simulink model "DC_DC_buck_Microgrid_sim_4"  (R2015a)
settings: Solver=ode23tb  StartTime=0.0  StopTime=0.05  MaxStep=1/fpwm/200  RelTol=1e-3
values from neighbouring files (symbols this model uses):
  Cf = 2*IoAVmin/(8*fpwm*DeltaVo*Vo)    (= 5.42534722222e-05)    [DC_DC_buck_Microgrid_1_2_3.m]    (also in DC_DC_buck_Microgrid_4.m = 2.71267361111e-05)
  Cf2 = 2*IoAVmin2/(8*fpwm2*DeltaVo2*Vo2)    (= 5.42534722222e-05)    [DC_DC_buck_Microgrid_4.m]
  deltaN = Vo/U    (= 0.48)    [DC_DC_buck_Microgrid_1_2_3.m]    (also in DC_DC_buck_Microgrid_4.m)
  fpwm = 10000    [DC_DC_buck_Microgrid_1_2_3.m]    (also in DC_DC_buck_Microgrid_4.m = 20000)
  fpwm2 = 10000    [DC_DC_buck_Microgrid_4.m]
  IoAVmin = Pomin/Vo    (= 2.08333333333)    [DC_DC_buck_Microgrid_1_2_3.m]    (also in DC_DC_buck_Microgrid_4.m)
  IoAVmin2 = Pomin2/Vo2    (= 2.08333333333)    [DC_DC_buck_Microgrid_4.m]
  Ios = (Pom-Pp-Pomin-Vo^2/Reqp)/Vo    [DC_DC_buck_Microgrid_1_2_3.m]    (also in DC_DC_buck_Microgrid_4.m = 15.625)
  kdv = -(Vomin-Vomax)/(Po-Pomin)    (= 0.00571428571429)    [DC_DC_buck_Microgrid_4.m]
  kdv2 = -(Vomin2-Vomax2)/(Po2-Pomin2)    (= 0.00333333333333)    [DC_DC_buck_Microgrid_4.m]
  Ki = 1/Tp    (= 153.646401213)    [DC_DC_buck_Microgrid_1_2_3.m]    (also in DC_DC_buck_Microgrid_4.m = 307.292802426)
  Ki2 = 1/Tp2    (= 76.8232006066)    [DC_DC_buck_Microgrid_4.m]
  Kiv = 1/Tpv    (= 2252.73933103)    [DC_DC_buck_Microgrid_1_2_3.m]    (also in DC_DC_buck_Microgrid_4.m = 4505.47866205)
  Kiv2 = 1/Tpv2    (= 3754.56555171)    [DC_DC_buck_Microgrid_4.m]
  Kp = Tz/Tp    (= 0.0678081650224)    [DC_DC_buck_Microgrid_1_2_3.m]    (also in DC_DC_buck_Microgrid_4.m)
  Kp2 = Tz2/Tp2    (= 0.0632538852821)    [DC_DC_buck_Microgrid_4.m]
  Kpv = Tzv/Tpv    (= 0.187728277586)    [DC_DC_buck_Microgrid_1_2_3.m]    (also in DC_DC_buck_Microgrid_4.m)
  Kpv2 = Tzv2/Tpv2    (= 0.187728277586)    [DC_DC_buck_Microgrid_4.m]
  Lf = 1.01*Vo*(1-deltamin)/(2*IoAVmin*fpwm)    (= 0.000677876869565)    [DC_DC_buck_Microgrid_1_2_3.m]    (also in DC_DC_buck_Microgrid_4.m = 0.000338938434783)
  Lf2 = 1.01*Vo2*(1-deltamin2)/(2*IoAVmin2*fpwm2)    (= 0.000758817391304)    [DC_DC_buck_Microgrid_4.m]
  Po = 1500    [DC_DC_buck_Microgrid_1_2_3.m]    (also in DC_DC_buck_Microgrid_4.m)
  Po2 = 2500    [DC_DC_buck_Microgrid_4.m]
  Pomin = 100    [DC_DC_buck_Microgrid_1_2_3.m]    (also in DC_DC_buck_Microgrid_4.m)
  Pomin2 = 100    [DC_DC_buck_Microgrid_4.m]
  Rdv = -(Vomin-Vomax)/(Imax-Imin)    (= 0.274285714286)    [DC_DC_buck_Microgrid_4.m]
  Rdv2 = -(Vomin2-Vomax2)/(Imax2-Imin2)    (= 0.16)    [DC_DC_buck_Microgrid_4.m]
  Req = Vo^2/Po    (= 1.536)    [DC_DC_buck_Microgrid_1_2_3.m]    (also in DC_DC_buck_Microgrid_4.m = 1.64571428571)
  Req2 = Vomin2^2/(Po2-Pomin2)    (= 0.96)    [DC_DC_buck_Microgrid_4.m]
  ri = 0.01    [DC_DC_buck_Microgrid_1_2_3.m]    (also in DC_DC_buck_Microgrid_4.m)
  ri2 = 0.005    [DC_DC_buck_Microgrid_4.m]
  rLine = 0.04    [DC_DC_buck_Microgrid_4.m]
  rLine2 = 0.04    [DC_DC_buck_Microgrid_4.m]
  Rmax = Vo^2/Pomin    (= 23.04)    [DC_DC_buck_Microgrid_1_2_3.m]    (also in DC_DC_buck_Microgrid_4.m)
  Rmax2 = Vo2^2/Pomin2    (= 23.04)    [DC_DC_buck_Microgrid_4.m]
  U = 100    [DC_DC_buck_Microgrid_1_2_3.m]    (also in DC_DC_buck_Microgrid_4.m)
  U2 = 120    [DC_DC_buck_Microgrid_4.m]
  ucmax = 1    [DC_DC_buck_Microgrid_1_2_3.m]    (also in DC_DC_buck_Microgrid_4.m)
  ucmax2 = 1    [DC_DC_buck_Microgrid_4.m]
  Vo = 48    [DC_DC_buck_Microgrid_1_2_3.m]    (also in DC_DC_buck_Microgrid_4.m)
  Vomax = 56    [DC_DC_buck_Microgrid_4.m]
  Vomin = Vo    (= 48)    [DC_DC_buck_Microgrid_4.m]
  Vomin2 = Vo    (= 48)    [DC_DC_buck_Microgrid_4.m]
libraries: powerlib x39, simulink x5, powerlib_meascontrol x4
settings Model: Creator=fern  LastModifiedBy=fern

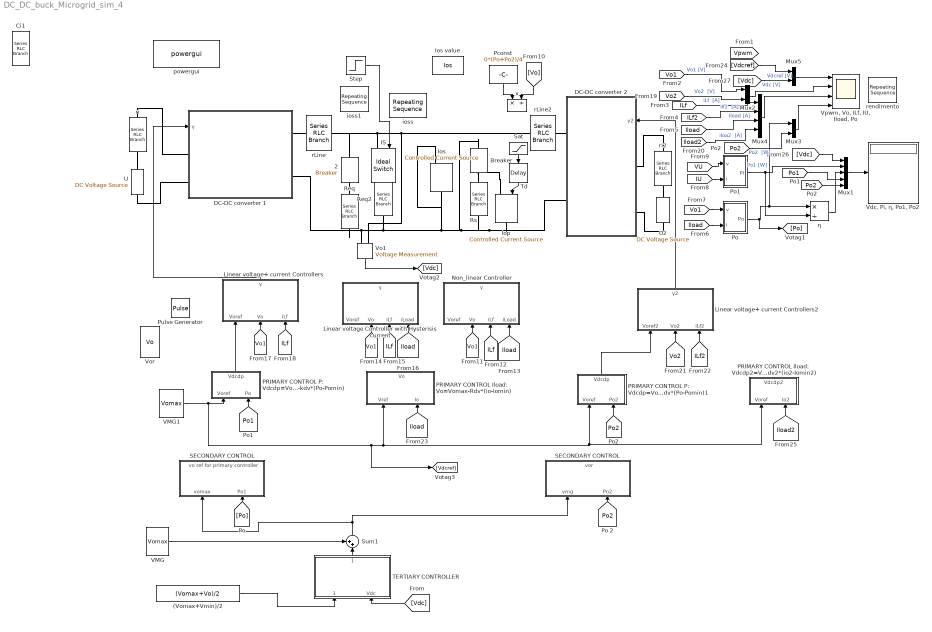
== system DC_DC_buck_Microgrid_sim_4 ==
  (Vomax+Vmin)/2 : Constant  Value=(Vomax+Vo)/2
  2 : powerlib/Elements/Breaker  InitialState=0  SwitchingTimes=[0.01]  External=off  BreakerResistance=0.01  SnubberResistance=Rs  SnubberCapacitance=Cs  Measurements=None  MoreParameters=on  NoBreakLoop=off
  Breaker : powerlib/Elements/Breaker  InitialState=0  SwitchingTimes=[0.04]  External=off  BreakerResistance=0.01  SnubberResistance=Rs  SnubberCapacitance=Cs  Measurements=None  MoreParameters=on  NoBreakLoop=off
  Ci1 : powerlib/Elements/Series RLC Branch  LConnTagsString=__new0  RConnTagsString=__new0  BranchType=C  Resistance=ri  Inductance=1e-6  SetiL0=off  InitialCurrent=4  Capacitance=100e-6  Setx0=on  InitialVoltage=U  Measurements=None
  DC-DC converter 1 : Subsystem
  DC-DC converter 2 : Subsystem
  IS : powerlib/Power Electronics/Ideal Switch  Ron=0.01  Lon=0  IC=0  Rs=Rs  Cs=Cs  Measurements=off
  Iop : powerlib/Electrical Sources/Controlled Current Source  Initialize=on  Source_Type=DC  Amplitude=0  Phase=0  Frequency=0  Measurements=None
  Ios : powerlib/Electrical Sources/Controlled Current Source  Initialize=on  Source_Type=DC  Amplitude=0  Phase=0  Frequency=0  Measurements=None
  Ios value : Constant  Value=Ios
  Linear voltage Controller with Hysterisis current : Subsystem
  Linear voltage+ current Controllers : Subsystem
  Linear voltage+ current Controllers2 : Subsystem
  Mux1 : Mux  Inputs=5
  Mux2 : Mux  Inputs=2
  Mux3 : Mux  Inputs=2
  Mux4 : Mux
  Mux5 : Mux  Inputs=2
  Non_linear Controller : Subsystem
  PRIMARY CONTROL Iload: Vdcdp2=Vomax2-Rdv2*(io2-Iomin2) : Subsystem
  PRIMARY CONTROL Iload: Vo=Vomax-Rdv*(io-Iomin) : Subsystem
  PRIMARY CONTROL P: Vdcdp=Vomax-kdv*(Po-Pomin) : Subsystem
  PRIMARY CONTROL P: Vdcdp=Vomax-kdv*(Po-Pomin)1 : Subsystem
  Pconst : Constant  Value=0*(Po+Po2)/4
  Po : Subsystem
  Po1 : Subsystem
  Pulse Generator : DiscretePulseGenerator  PulseType=Time based  Period=1/fpwm  PulseWidth=deltaN*100
  Req : powerlib/Elements/Series RLC Branch  LConnTagsString=__new0  RConnTagsString=__new0  BranchType=R  Resistance=Req  Inductance=500e-3  SetiL0=on  InitialCurrent=43  Capacitance=[]  Setx0=off  InitialVoltage=0  Measurements=None
  Req2 : powerlib/Elements/Series RLC Branch  LConnTagsString=__new0  RConnTagsString=__new0  BranchType=R  Resistance=Req2  Inductance=500e-3  SetiL0=on  InitialCurrent=43  Capacitance=[]  Setx0=off  InitialVoltage=0  Measurements=None
  Rs : powerlib/Elements/Series RLC Branch  LConnTagsString=__new0  RConnTagsString=__new0  BranchType=R  Resistance=1000*Rmax  Inductance=500e-3  SetiL0=on  InitialCurrent=43  Capacitance=[]  Setx0=off  InitialVoltage=0  Measurements=None
  "SECONDARY CONTROL " : Subsystem
  "SECONDARY CONTROL  " : Subsystem
  Sat : Saturate  UpperLimit=30  LowerLimit=0
  Step : Step  Time=0.02  SampleTime=0
  Sum1 : Sum  Inputs=++|
  TERTIARY CONTROLLER : Subsystem
  Td : TransportDelay  DelayTime=1/(2*fpwm)  BufferSize=2048
  U : powerlib/Electrical Sources/DC Voltage Source  Description=source block  Amplitude=U  Measurements=None
      settings: AttributesFormatString=\n
  U2 : powerlib/Electrical Sources/DC Voltage Source  Description=source block  Amplitude=U2  Measurements=None
      settings: AttributesFormatString=\n
  VMG : Constant  Value=Vomax
  VMG1 : Constant  Value=Vomax
  "Vdc, Pi, η, Po1, Po2" : Display
      settings: Decimation=1000
  Vo1 : powerlib/Measurements/Voltage Measurement  Tag=PoWeRsYsTeMmEaSuReMeNt  PhasorSimulation=off  OutputType=Complex  PSBequivalent=0
  Vor : Constant  Value=Vo
  "Vpwm, Vo, ILf, IU, Iload, Po" : Scope  NumInputPorts=4
      settings: ShowLegends=on  TimeRange=0.0001950120476463327  YMin=55.4~55.3~0~125  YMax=56.3~56.3~5~145  SaveName=psbconverter_str  SampleTime=1/50/512
  ioss : simulink/Sources/Repeating Sequence  rep_seq_t="[0 0.01  0.09 0.1]"  rep_seq_y=[0 0 (Po+Po2-Pomin-Pomin2)/Vomin (Po+Po2-Pomin-Pomin2)/Vomin]
  ioss1 : simulink/Sources/Repeating Sequence  rep_seq_t="[0 0.0149 0.015  0.035 0.03501 0.1]"  rep_seq_y=[0 0 1 1 0 0]
  powergui : powerlib/powergui  Priority=2  SimulationMode=Continuous  SolverType=Tustin/Backward Euler (TBE)  SampleTime=0  frequency=60  SPID=off  DisableSnubberDevices=off  DisableRonSwitches=off  DisableVfSwitches=off  SwTol=0  DisplayEquations=off  Interpol=off  methode=off  Ts=0  FunctionMessages=off  echomessages=off  HookPort=off  EnableUseOfTLC=off  x0status=blocks  frequencyindice=0  Pbase=100e6  ErrMax=1e-4  Iterations=50  UnitsV=kV  UnitsW=MW  buscounter=0  RestoreLinks=warning  ResistiveCurrentMeasurement=off  Frange=[0:2:500]  Ylog=off  Xlog=on  ShowGrid=off  save=off  variable=ZData  structure=psbconverter_str  ZoomFFT=on  StartTime=0.1-2/60  cycles=2  DisplayStyle=off  fundamental=60  FreqAxis=on  MaxFrequency=2000  frequencyindicesteady=1  RmsSteady=1  display=off
  rLine : powerlib/Elements/Series RLC Branch  LConnTagsString=__new0  RConnTagsString=__new0  BranchType=R  Resistance=rLine  Inductance=1e-6  SetiL0=off  InitialCurrent=4  Capacitance=[]  Setx0=off  InitialVoltage=0  Measurements=None
  rLine2 : powerlib/Elements/Series RLC Branch  LConnTagsString=__new0  RConnTagsString=__new0  BranchType=R  Resistance=rLine2  Inductance=1e-6  SetiL0=off  InitialCurrent=4  Capacitance=[]  Setx0=off  InitialVoltage=0  Measurements=None
  rendimento : simulink/Sources/Repeating Sequence  rep_seq_t=[0 0.1]  rep_seq_y=[0 30]
  ri : powerlib/Elements/Series RLC Branch  LConnTagsString=__new0  RConnTagsString=__new0  BranchType=R  Resistance=ri  Inductance=1e-6  SetiL0=off  InitialCurrent=4  Capacitance=[]  Setx0=off  InitialVoltage=0  Measurements=None
  ri2 : powerlib/Elements/Series RLC Branch  LConnTagsString=__new0  RConnTagsString=__new0  BranchType=R  Resistance=ri2  Inductance=1e-6  SetiL0=off  InitialCurrent=4  Capacitance=[]  Setx0=off  InitialVoltage=0  Measurements=None
  x : Product  Inputs=*/
  η : Product  Inputs=*/
  wires:
  Pconst/1 -> x/1
  Mux2/1 -> "Vpwm, Vo, ILf, IU, Iload, Po"/2
  [ILf] -> Mux4/1  "iLf  [A]"
  [Iload] -> Mux4/3  "Iload [A]"
  Mux4/1 -> "Vpwm, Vo, ILf, IU, Iload, Po"/3
  [Vo1] -> Po/1(v)
  [Iload] -> Po/2(i)
  Po/1(Po) -> [Po], Mux3/1, η/1  "Po1 [W]"
  Mux1/1 -> "Vdc, Pi, η, Po1, Po2"/1
  [VU] -> Po1/1(v)
  [IU] -> Po1/2(i)
  Po1/1(Pi) -> η/2, Mux1/2
  [Vo] -> x/2
  Sat/1 -> Td/1
  [Iload] -> Linear voltage Controller with Hysterisis current/4(iLoad)
  [ILf] -> Linear voltage Controller with Hysterisis current/3(iLf)
  [Vo1] -> Linear voltage Controller with Hysterisis current/2(Vo)
  [Vo1] -> Non_linear Controller/2(Vo)
  [ILf] -> Non_linear Controller/3(iLf)
  [Iload] -> Non_linear Controller/4(iLoad)
  [ILf] -> Linear voltage+ current Controllers/3(iLf)
  [Vo1] -> Linear voltage+ current Controllers/2(Vo)
  [Vo1] -> Mux2/1  "Vo1 [V]"
  Mux3/1 -> "Vpwm, Vo, ILf, IU, Iload, Po"/4
  [Vo2] -> Linear voltage+ current Controllers2/2(Vo2)
  [ILf2] -> Linear voltage+ current Controllers2/3(iLf2)
  [Po2] -> PRIMARY CONTROL P: Vdcdp=Vomax-kdv*(Po-Pomin)1/2(Po2)
  [Po1] -> PRIMARY CONTROL P: Vdcdp=Vomax-kdv*(Po-Pomin)/2(Po)
  [Iload] -> PRIMARY CONTROL Iload: Vo=Vomax-Rdv*(io-Iomin)/2(Io)
  Vo1/1 -> [Vdc]
  η/1 -> Mux1/3
  [Po2] -> Mux1/5
  [Po1] -> Mux1/4
  [Iload2] -> PRIMARY CONTROL Iload: Vdcdp2=Vomax2-Rdv2*(io2-Iomin2)/2(Io2)
  [Po] -> "SECONDARY CONTROL "/2(Po1)
  [Po2] -> "SECONDARY CONTROL  "/2(Po2)
  (Vomax+Vmin)/2/1 -> TERTIARY CONTROLLER/1((Vomax+Vmin)/2)
  [Vdc] -> TERTIARY CONTROLLER/2(Vdc)
  Td/1 -> Iop/1
  [Vdc] -> Mux1/1
  Step/1 -> IS/1
  VMG/1 -> Sum1/1
  Mux5/1 -> "Vpwm, Vo, ILf, IU, Iload, Po"/1
  [Vdcref] -> Mux5/1  "Vdcref [V]"
  [Vdc] -> Mux5/2  "Vdc [V]"
  TERTIARY CONTROLLER/1(Voref for secondary controller) -> Sum1/2
  Linear voltage+ current Controllers/1(γ) -> DC-DC converter 1/1(γ)
  Linear voltage+ current Controllers2/1(γ2) -> DC-DC converter 2/1(γ2)
  Sum1/1 -> "SECONDARY CONTROL "/1(vomax), "SECONDARY CONTROL  "/1(vmg)
  [Vo2] -> Mux2/2  "Vo2  [V]"
  [ILf2] -> Mux4/2  "ilf2  [A]"
  [Iload2] -> Mux4/4  "iloa2  [A]"
  [Po2] -> Mux3/2  "Po2  [W]"
  VMG1/1 -> [Vdcref], PRIMARY CONTROL Iload: Vo=Vomax-Rdv*(io-Iomin)/1(Vref), PRIMARY CONTROL Iload: Vdcdp2=Vomax2-Rdv2*(io2-Iomin2)/1(Voref), PRIMARY CONTROL P: Vdcdp=Vomax-kdv*(Po-Pomin)1/1(Voref), PRIMARY CONTROL P: Vdcdp=Vomax-kdv*(Po-Pomin)/1(Voref)
  PRIMARY CONTROL P: Vdcdp=Vomax-kdv*(Po-Pomin)1/1(Vdcdp) -> Linear voltage+ current Controllers2/1(Voref2)
  PRIMARY CONTROL P: Vdcdp=Vomax-kdv*(Po-Pomin)/1(Vdcdp) -> Linear voltage+ current Controllers/1(Voref)
  connections:
  U/RConn1 -- ri/RConn1
  rLine2/RConn1 -- Vo1/LConn1 -- 2/LConn1 -- rLine/RConn1 -- IS/LConn1
  rLine2/LConn1 -- DC-DC converter 2/RConn1
  2/RConn1 -- Req/LConn1
  IS/RConn1 -- Req2/LConn1
  Rs/LConn1 -- Breaker/RConn1 -- Iop/LConn1
  Req2/RConn1 -- Breaker/LConn1 -- DC-DC converter 2/RConn2 -- Iop/RConn1 -- Rs/RConn1 -- Ios/LConn1 -- Ios/RConn1 -- Vo1/LConn2 -- DC-DC converter 1/RConn2 -- Req/RConn1
  DC-DC converter 1/LConn1 -- ri/LConn1
  DC-DC converter 1/LConn2 -- U/LConn1
  DC-DC converter 1/RConn1 -- rLine/LConn1
  U2/RConn1 -- ri2/RConn1
  ri2/LConn1 -- DC-DC converter 2/LConn1
  U2/LConn1 -- DC-DC converter 2/LConn2

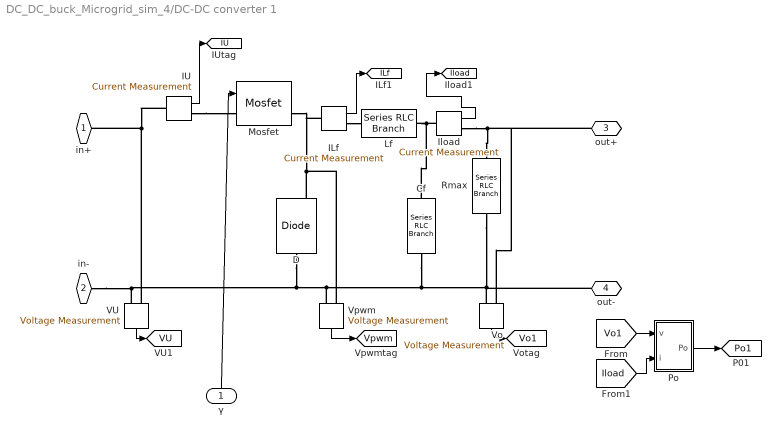
== system DC_DC_buck_Microgrid_sim_4/DC-DC converter 1 ==
  γ : Inport
  Cf : powerlib/Elements/Series RLC Branch  LConnTagsString=__new0  RConnTagsString=__new0  BranchType=C  Resistance=ri  Inductance=Lf  SetiL0=on  InitialCurrent=IoAVmin  Capacitance=Cf  Setx0=on  InitialVoltage=Vo  Measurements=None
  D : powerlib/Power Electronics/Diode  Ron=Ron  Lon=0  Vf=Vd  IC=0  UseSnubber=off  Rs=Rs  Cs=Cs  Measurements=on
  ILf : powerlib/Measurements/Current Measurement  PhasorSimulation=off  OutputType=Complex  PSBequivalent=0
  IU : powerlib/Measurements/Current Measurement  PhasorSimulation=off  OutputType=Complex  PSBequivalent=0
  Iload : powerlib/Measurements/Current Measurement  PhasorSimulation=off  OutputType=Complex  PSBequivalent=0
  Lf : powerlib/Elements/Series RLC Branch  LConnTagsString=__new0  RConnTagsString=__new0  BranchType=L  Resistance=ri  Inductance=Lf  SetiL0=on  InitialCurrent=IoAVmin  Capacitance=[]  Setx0=off  InitialVoltage=0  Measurements=None
  Mosfet : powerlib/Power Electronics/Mosfet  Ron=Rdson  Lon=0  Rd=Rdson  Vfd=0  IC=0  Rs=Rs  Cs=Cs  Measurements=on
  Po : Subsystem
  Rmax : powerlib/Elements/Series RLC Branch  LConnTagsString=__new0  RConnTagsString=__new0  BranchType=R  Resistance=Rmax  Inductance=500e-3  SetiL0=on  InitialCurrent=43  Capacitance=[]  Setx0=off  InitialVoltage=0  Measurements=None
  VU : powerlib/Measurements/Voltage Measurement  Tag=PoWeRsYsTeMmEaSuReMeNt  PhasorSimulation=off  OutputType=Complex  PSBequivalent=0
  Vo : powerlib/Measurements/Voltage Measurement  Tag=PoWeRsYsTeMmEaSuReMeNt  PhasorSimulation=off  OutputType=Complex  PSBequivalent=0
  Vpwm : powerlib/Measurements/Voltage Measurement  Tag=PoWeRsYsTeMmEaSuReMeNt  PhasorSimulation=off  OutputType=Complex  PSBequivalent=0
  in+ : PMIOPort  Port=1  Side=Left
  in- : PMIOPort  Port=2  Side=Left
  out+ : PMIOPort  Port=3  Side=Right
  out- : PMIOPort  Port=4  Side=Right
  tag scope: ILf=global, IU=global, Iload=global, Po1=global, VU=global, Vo1=global, Vpwm=global
  wires:
  Iload/1 -> [Iload]
  Vo/1 -> [Vo1]
  Vpwm/1 -> [Vpwm]
  IU/1 -> [IU]
  VU/1 -> [VU]
  ILf/1 -> [ILf]
  γ/1 -> Mosfet/1
  [Vo1] -> Po/1(v)
  [Iload] -> Po/2(i)
  Po/1(Po) -> [Po1]
  connections:
  VU/LConn2 -- D/LConn1 -- Vpwm/LConn2 -- Cf/RConn1 -- out-/RConn1 -- Vo/LConn2 -- Rmax/RConn1 -- in-/RConn1
  D/RConn1 -- Mosfet/RConn1 -- ILf/LConn1 -- Vpwm/LConn1
  VU/LConn1 -- IU/LConn1 -- in+/RConn1
  Cf/LConn1 -- Iload/LConn1 -- Lf/RConn1
  ILf/RConn1 -- Lf/LConn1
  IU/RConn1 -- Mosfet/LConn1
  Iload/RConn1 -- out+/RConn1 -- Vo/LConn1 -- Rmax/LConn1

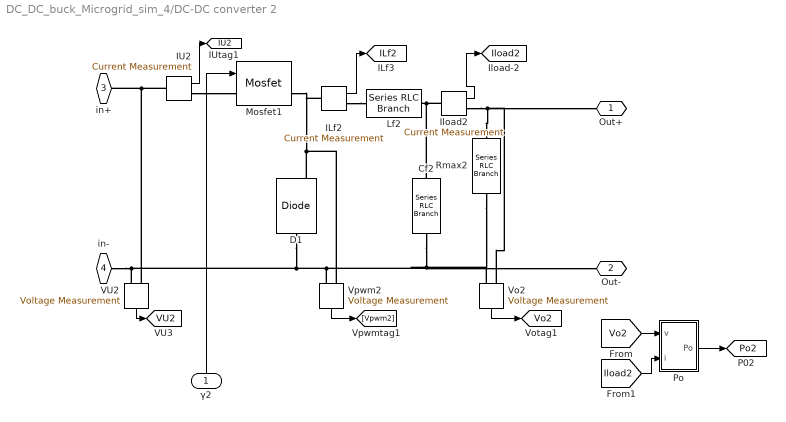
== system DC_DC_buck_Microgrid_sim_4/DC-DC converter 2 ==
  γ2 : Inport
  Cf2 : powerlib/Elements/Series RLC Branch  LConnTagsString=__new0  RConnTagsString=__new0  BranchType=C  Resistance=ri  Inductance=Lf  SetiL0=on  InitialCurrent=IoAVmin  Capacitance=Cf2  Setx0=on  InitialVoltage=Vo  Measurements=None
  D1 : powerlib/Power Electronics/Diode  Ron=Ron2  Lon=0  Vf=Vd2  IC=0  UseSnubber=off  Rs=Rs2  Cs=Cs2  Measurements=on
  ILf2 : powerlib/Measurements/Current Measurement  PhasorSimulation=off  OutputType=Complex  PSBequivalent=0
  IU2 : powerlib/Measurements/Current Measurement  PhasorSimulation=off  OutputType=Complex  PSBequivalent=0
  Iload2 : powerlib/Measurements/Current Measurement  PhasorSimulation=off  OutputType=Complex  PSBequivalent=0
  Lf2 : powerlib/Elements/Series RLC Branch  LConnTagsString=__new0  RConnTagsString=__new0  BranchType=L  Resistance=ri  Inductance=Lf2  SetiL0=off  InitialCurrent=IoAV2min  Capacitance=[]  Setx0=off  InitialVoltage=0  Measurements=None
  Mosfet1 : powerlib/Power Electronics/Mosfet  Ron=Rdson2  Lon=0  Rd=Rdson2  Vfd=0  IC=0  Rs=Rs2  Cs=Cs2  Measurements=on
  Po : Subsystem
  Rmax2 : powerlib/Elements/Series RLC Branch  LConnTagsString=__new0  RConnTagsString=__new0  BranchType=R  Resistance=Rmax2  Inductance=500e-3  SetiL0=on  InitialCurrent=43  Capacitance=[]  Setx0=off  InitialVoltage=0  Measurements=None
  VU2 : powerlib/Measurements/Voltage Measurement  Tag=PoWeRsYsTeMmEaSuReMeNt  PhasorSimulation=off  OutputType=Complex  PSBequivalent=0
  Vo2 : powerlib/Measurements/Voltage Measurement  Tag=PoWeRsYsTeMmEaSuReMeNt  PhasorSimulation=off  OutputType=Complex  PSBequivalent=0
  Vpwm2 : powerlib/Measurements/Voltage Measurement  Tag=PoWeRsYsTeMmEaSuReMeNt  PhasorSimulation=off  OutputType=Complex  PSBequivalent=0
  Out+ : PMIOPort  Port=1  Side=Right
  Out- : PMIOPort  Port=2  Side=Right
  in+ : PMIOPort  Port=3  Side=Left
  in- : PMIOPort  Port=4  Side=Left
  tag scope: ILf2=global, IU2=global, Iload2=global, Po2=global, VU2=global, Vo2=global
  wires:
  VU2/1 -> [VU2]
  IU2/1 -> [IU2]
  Iload2/1 -> [Iload2]
  Vo2/1 -> [Vo2]
  ILf2/1 -> [ILf2]
  γ2/1 -> Mosfet1/1
  Vpwm2/1 -> [Vpwm2]
  [Vo2] -> Po/1(v)
  [Iload2] -> Po/2(i)
  Po/1(Po) -> [Po2]
  connections:
  D1/RConn1 -- Vpwm2/LConn1 -- ILf2/LConn1 -- Mosfet1/RConn1
  D1/LConn1 -- VU2/LConn2 -- in-/RConn1 -- Vpwm2/LConn2 -- Cf2/RConn1 -- Out-/RConn1 -- Vo2/LConn2 -- Rmax2/RConn1
  VU2/LConn1 -- in+/RConn1 -- IU2/LConn1
  Cf2/LConn1 -- Iload2/LConn1 -- Lf2/RConn1
  IU2/RConn1 -- Mosfet1/LConn1
  ILf2/RConn1 -- Lf2/LConn1
  Iload2/RConn1 -- Out+/RConn1 -- Vo2/LConn1 -- Rmax2/LConn1

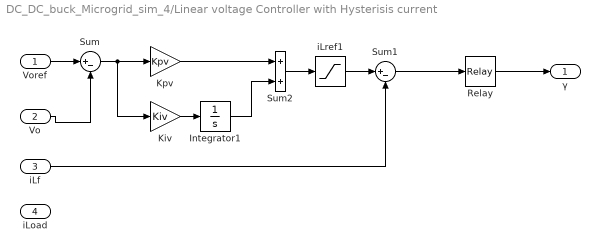
== system DC_DC_buck_Microgrid_sim_4/Linear voltage Controller with Hysterisis current ==
  Voref : Inport
  Vo : Inport  Port=2
  iLf : Inport  Port=3
  iLoad : Inport  Port=4
  Integrator1 : Integrator  LimitOutput=on  UpperSaturationLimit=60  LowerSaturationLimit=-60
  Kiv : Gain  Gain=Kiv
  Kpv : Gain  Gain=Kpv
  Relay : Relay  OnSwitchValue=IoAVmin/2  OffSwitchValue=-IoAVmin/2
  Sum : Sum  Inputs=|+-
  Sum1 : Sum  Inputs=|+-
  Sum2 : Sum
  iLref1 : Saturate  UpperLimit=60  LowerLimit=0
  γ : Outport
  wires:
  Kpv/1 -> Sum2/1
  Sum1/1 -> Relay/1
  Sum/1 -> Kiv/1, Kpv/1
  Vo/1 -> Sum/2
  Voref/1 -> Sum/1
  Relay/1 -> γ/1
  Sum2/1 -> iLref1/1
  iLf/1 -> Sum1/2
  Kiv/1 -> Integrator1/1
  Integrator1/1 -> Sum2/2
  iLref1/1 -> Sum1/1

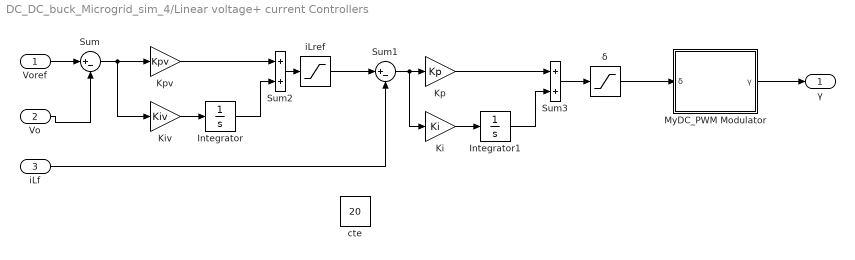
== system DC_DC_buck_Microgrid_sim_4/Linear voltage+ current Controllers ==
  Voref : Inport
  Vo : Inport  Port=2
  iLf : Inport  Port=3
  Integrator : Integrator  LimitOutput=on  UpperSaturationLimit=1.3*Po/Vomin  LowerSaturationLimit=-1.3*Po/Vomin
  Integrator1 : Integrator  LimitOutput=on  UpperSaturationLimit=1  LowerSaturationLimit=-1
  Ki : Gain  Gain=Ki
  Kiv : Gain  Gain=Kiv
  Kp : Gain  Gain=Kp
  Kpv : Gain  Gain=Kpv
  MyDC_PWM Modulator : Subsystem
  Sum : Sum  Inputs=|+-
  Sum1 : Sum  Inputs=|+-
  Sum2 : Sum
  Sum3 : Sum
  cte : Constant  Value=20
  iLref : Saturate  UpperLimit=1.3*Po/Vomin  LowerLimit=0
  δ : Saturate  UpperLimit=0.99  LowerLimit=0.01
  γ : Outport
  wires:
  Integrator/1 -> Sum2/2
  Kiv/1 -> Integrator/1
  iLf/1 -> Sum1/2
  Sum2/1 -> iLref/1
  Voref/1 -> Sum/1
  Vo/1 -> Sum/2
  Sum/1 -> Kpv/1, Kiv/1
  Kpv/1 -> Sum2/1
  Integrator1/1 -> Sum3/2
  Ki/1 -> Integrator1/1
  Sum3/1 -> δ/1
  Sum1/1 -> Kp/1, Ki/1
  Kp/1 -> Sum3/1
  iLref/1 -> Sum1/1
  δ/1 -> MyDC_PWM Modulator/1(δ)
  MyDC_PWM Modulator/1(γ) -> γ/1

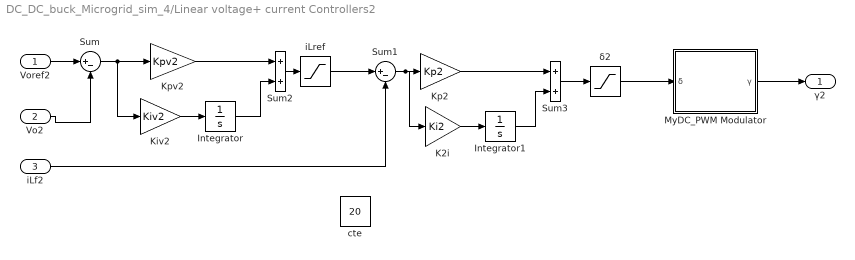
== system DC_DC_buck_Microgrid_sim_4/Linear voltage+ current Controllers2 ==
  Voref2 : Inport
  Vo2 : Inport  Port=2
  iLf2 : Inport  Port=3
  Integrator : Integrator  LimitOutput=on  UpperSaturationLimit=1.3*Po2/Vomin2  LowerSaturationLimit=-1.3*Po2/Vomin2
  Integrator1 : Integrator  LimitOutput=on  UpperSaturationLimit=1  LowerSaturationLimit=-1
  K2i : Gain  Gain=Ki2
  Kiv2 : Gain  Gain=Kiv2
  Kp2 : Gain  Gain=Kp2
  Kpv2 : Gain  Gain=Kpv2
  MyDC_PWM Modulator : Subsystem
  Sum : Sum  Inputs=|+-
  Sum1 : Sum  Inputs=|+-
  Sum2 : Sum
  Sum3 : Sum
  cte : Constant  Value=20
  iLref : Saturate  UpperLimit=1.3*Po2/Vomin2  LowerLimit=0
  δ2 : Saturate  UpperLimit=0.99  LowerLimit=0.01
  γ2 : Outport
  wires:
  MyDC_PWM Modulator/1(γ) -> γ2/1
  δ2/1 -> MyDC_PWM Modulator/1(δ)
  iLref/1 -> Sum1/1
  Kp2/1 -> Sum3/1
  Sum1/1 -> K2i/1, Kp2/1
  Sum3/1 -> δ2/1
  K2i/1 -> Integrator1/1
  Integrator1/1 -> Sum3/2
  Kpv2/1 -> Sum2/1
  Sum/1 -> Kiv2/1, Kpv2/1
  Vo2/1 -> Sum/2
  Voref2/1 -> Sum/1
  Sum2/1 -> iLref/1
  iLf2/1 -> Sum1/2
  Kiv2/1 -> Integrator/1
  Integrator/1 -> Sum2/2

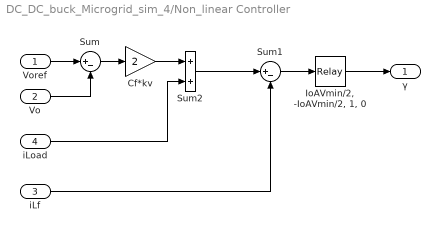
== system DC_DC_buck_Microgrid_sim_4/Non_linear Controller ==
  Voref : Inport
  Vo : Inport  Port=2
  iLf : Inport  Port=3
  iLoad : Inport  Port=4
  Cf*kv : Gain  Gain=2
  "IoAVmin/2, -IoAVmin/2, 1, 0" : Relay  OnSwitchValue=IoAVmin/2  OffSwitchValue=-IoAVmin/2
  Sum : Sum  Inputs=|+-
  Sum1 : Sum  Inputs=|+-
  Sum2 : Sum
  γ : Outport
  wires:
  "IoAVmin/2, -IoAVmin/2, 1, 0"/1 -> γ/1
  Voref/1 -> Sum/1
  Vo/1 -> Sum/2
  Sum/1 -> Cf*kv/1
  iLf/1 -> Sum1/2
  Sum1/1 -> "IoAVmin/2, -IoAVmin/2, 1, 0"/1
  Cf*kv/1 -> Sum2/1
  Sum2/1 -> Sum1/1
  iLoad/1 -> Sum2/2

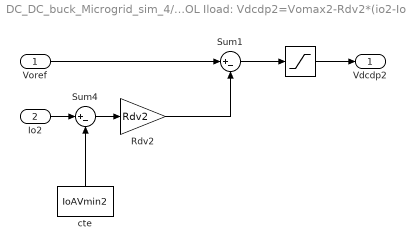
== system DC_DC_buck_Microgrid_sim_4/PRIMARY CONTROL Iload: Vdcdp2=Vomax2-Rdv2*(io2-Iomin2) ==
  Voref : Inport
  Io2 : Inport  Port=2
  " " : Saturate  UpperLimit=Vomax+1  LowerLimit=Vomin-1
  Rdv2 : Gain  Gain=Rdv2
  Sum1 : Sum  Inputs=|+-
  Sum4 : Sum  Inputs=|+-
  cte : Constant  Value=IoAVmin2
  Vdcdp2 : Outport
  wires:
  Sum1/1 -> " "/1
  Voref/1 -> Sum1/1
  Io2/1 -> Sum4/1
  cte/1 -> Sum4/2
  Sum4/1 -> Rdv2/1
  " "/1 -> Vdcdp2/1
  Rdv2/1 -> Sum1/2

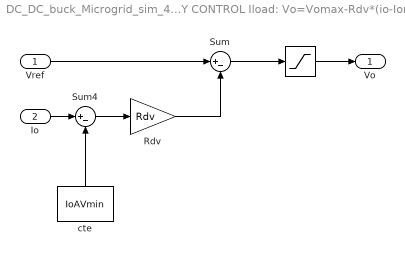
== system DC_DC_buck_Microgrid_sim_4/PRIMARY CONTROL Iload: Vo=Vomax-Rdv*(io-Iomin) ==
  Vref : Inport
  Io : Inport  Port=2
  " " : Saturate  UpperLimit=Vomax+1  LowerLimit=Vomin-1
  Rdv : Gain  Gain=Rdv
  Sum : Sum  Inputs=|+-
  Sum4 : Sum  Inputs=|+-
  cte : Constant  Value=IoAVmin
  Vo : Outport
  wires:
  " "/1 -> Vo/1
  Rdv/1 -> Sum/2
  Sum4/1 -> Rdv/1
  cte/1 -> Sum4/2
  Io/1 -> Sum4/1
  Vref/1 -> Sum/1
  Sum/1 -> " "/1

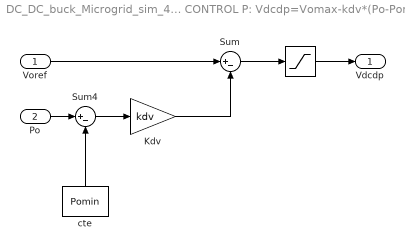
== system DC_DC_buck_Microgrid_sim_4/PRIMARY CONTROL P: Vdcdp=Vomax-kdv*(Po-Pomin) ==
  Voref : Inport
  Po : Inport  Port=2
  " " : Saturate  UpperLimit=Vomax+1  LowerLimit=Vomin-1
  Kdv : Gain  Gain=kdv
  Sum : Sum  Inputs=|+-
  Sum4 : Sum  Inputs=|+-
  cte : Constant  Value=Pomin
  Vdcdp : Outport
  wires:
  Sum/1 -> " "/1
  Voref/1 -> Sum/1
  Po/1 -> Sum4/1
  cte/1 -> Sum4/2
  Sum4/1 -> Kdv/1
  Kdv/1 -> Sum/2
  " "/1 -> Vdcdp/1

== system DC_DC_buck_Microgrid_sim_4/PRIMARY CONTROL P: Vdcdp=Vomax-kdv*(Po-Pomin)1 ==
  Voref : Inport
  Po2 : Inport  Port=2
  " " : Saturate  UpperLimit=Vomax+1  LowerLimit=Vomin-1
  Kdv2 : Gain  Gain=kdv2
  Sum : Sum  Inputs=|+-
  Sum4 : Sum  Inputs=|+-
  cte : Constant  Value=Pomin2
  Vdcdp : Outport
  wires:
  " "/1 -> Vdcdp/1
  Sum4/1 -> Kdv2/1
  cte/1 -> Sum4/2
  Po2/1 -> Sum4/1
  Voref/1 -> Sum/1
  Sum/1 -> " "/1
  Kdv2/1 -> Sum/2

== system DC_DC_buck_Microgrid_sim_4/Po ==
  v : Inport
  i : Inport  Port=2
  Mean : powerlib_meascontrol/Measurements/Mean  Freq=fpwm/10  Vinit=100  Ts=0
  x : Product  Inputs=**
  Po : Outport
  wires:
  x/1 -> Mean/1
  v/1 -> x/1
  i/1 -> x/2
  Mean/1 -> Po/1

== system DC_DC_buck_Microgrid_sim_4/Po1 ==
  v : Inport
  i : Inport  Port=2
  Mean : powerlib_meascontrol/Measurements/Mean  Freq=fpwm/10  Vinit=110  Ts=0
  x : Product  Inputs=**
  Pi : Outport
  wires:
  Mean/1 -> Pi/1
  i/1 -> x/2
  v/1 -> x/1
  x/1 -> Mean/1

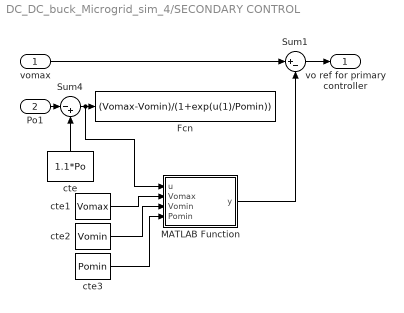
== system DC_DC_buck_Microgrid_sim_4/SECONDARY CONTROL  ==
  vomax : Inport
  Po1 : Inport  Port=2
  Fcn : Fcn  Expr=(Vomax-Vomin)/(1+exp(u(1)/Pomin))
  MATLAB Function : MATLAB Function  TreatAsAtomicUnit=on
  Sum1 : Sum  Inputs=|+-
  Sum4 : Sum  Inputs=|-+
  cte : Constant  Value=1.1*Po
  cte1 : Constant  Value=Vomax
  cte2 : Constant  Value=Vomin
  cte3 : Constant  Value=Pomin
  vo ref for primary controller : Outport
  wires:
  cte/1 -> Sum4/2
  Po1/1 -> Sum4/1
  Sum4/1 -> MATLAB Function/1(u), Fcn/1
  Sum1/1 -> vo ref for primary controller/1
  vomax/1 -> Sum1/1
  cte1/1 -> MATLAB Function/2(Vomax)
  cte2/1 -> MATLAB Function/3(Vomin)
  cte3/1 -> MATLAB Function/4(Pomin)
  MATLAB Function/1(y) -> Sum1/2

== system DC_DC_buck_Microgrid_sim_4/SECONDARY CONTROL   ==
  vmg : Inport
  Po2 : Inport  Port=2
  Fcn : Fcn  Expr=(Vomax-Vomin)/(1+exp(u(1)/Pomin2))
  Sum1 : Sum  Inputs=|+-
  Sum4 : Sum  Inputs=|-+
  cte : Constant  Value=1.1*Po2
  vor : Outport
  wires:
  Sum1/1 -> vor/1
  Po2/1 -> Sum4/1
  cte/1 -> Sum4/2
  Sum4/1 -> Fcn/1
  Fcn/1 -> Sum1/2
  vmg/1 -> Sum1/1

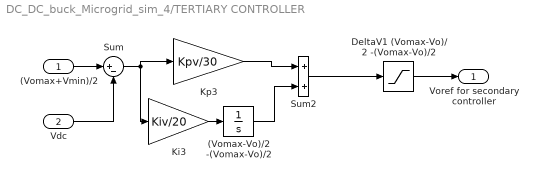
== system DC_DC_buck_Microgrid_sim_4/TERTIARY CONTROLLER ==
  (Vomax+Vmin)/2 : Inport
  Vdc : Inport  Port=2
  (Vomax-Vo)/2 -(Vomax-Vo)/2 : Integrator  LimitOutput=on  UpperSaturationLimit=(Vomax-Vo)/2  LowerSaturationLimit=-(Vomax-Vo)
  DeltaV1 (Vomax-Vo)/2 -(Vomax-Vo)/2 : Saturate  UpperLimit=(Vomax-Vo)/2  LowerLimit=-(Vomax-Vo)/2
  Ki3 : Gain  Gain=Kiv/20
  Kp3 : Gain  Gain=Kpv/30
  Sum : Sum  Inputs=|+-
  Sum2 : Sum
  Voref for secondary controller : Outport
  wires:
  DeltaV1 (Vomax-Vo)/2 -(Vomax-Vo)/2/1 -> Voref for secondary controller/1
  (Vomax-Vo)/2 -(Vomax-Vo)/2/1 -> Sum2/2
  Ki3/1 -> (Vomax-Vo)/2 -(Vomax-Vo)/2/1
  Sum2/1 -> DeltaV1 (Vomax-Vo)/2 -(Vomax-Vo)/2/1
  (Vomax+Vmin)/2/1 -> Sum/1
  Vdc/1 -> Sum/2
  Sum/1 -> Kp3/1, Ki3/1
  Kp3/1 -> Sum2/1

== system DC_DC_buck_Microgrid_sim_4/DC-DC converter 1/Po ==
  v : Inport
  i : Inport  Port=2
  Mean : powerlib_meascontrol/Measurements/Mean  Freq=fpwm/10  Vinit=100  Ts=0
  x : Product  Inputs=**
  Po : Outport
  wires:
  x/1 -> Mean/1
  v/1 -> x/1
  i/1 -> x/2
  Mean/1 -> Po/1

== system DC_DC_buck_Microgrid_sim_4/DC-DC converter 2/Po ==
  v : Inport
  i : Inport  Port=2
  Mean : powerlib_meascontrol/Measurements/Mean  Freq=fpwm/10  Vinit=100  Ts=0
  x : Product  Inputs=**
  Po : Outport
  wires:
  x/1 -> Mean/1
  v/1 -> x/1
  i/1 -> x/2
  Mean/1 -> Po/1

== system DC_DC_buck_Microgrid_sim_4/Linear voltage+ current Controllers/MyDC_PWM Modulator ==
  δ : Inport
  Relay : Relay  OnSwitchValue=0.01  OffSwitchValue=-0.01
  Sum4 : Sum  Inputs=|+-
  r(t) : simulink/Sources/Repeating Sequence  rep_seq_t=[0 1/fpwm]  rep_seq_y=[0 ucmax]
  γ : Outport
  wires:
  Relay/1 -> γ/1
  r(t)/1 -> Sum4/2
  Sum4/1 -> Relay/1
  δ/1 -> Sum4/1

== system DC_DC_buck_Microgrid_sim_4/Linear voltage+ current Controllers2/MyDC_PWM Modulator ==
  δ : Inport
  Relay : Relay  OnSwitchValue=0.01  OffSwitchValue=-0.01
  Sum4 : Sum  Inputs=|+-
  r(t) : simulink/Sources/Repeating Sequence  rep_seq_t=[0 1/fpwm2]  rep_seq_y=[0 ucmax2]
  γ : Outport
  wires:
  δ/1 -> Sum4/1
  Sum4/1 -> Relay/1
  r(t)/1 -> Sum4/2
  Relay/1 -> γ/1

== matlab function DC_DC_buck_Microgrid_sim_4/SECONDARY CONTROL /MATLAB Function ==
  data: u input; y output; Vomax input; Vomin input; Pomin input
function y = fcn(u, Vomax, Vomin, Pomin)
%#codegen

y = (Vomax-Vomin)/(1+exp(u/Pomin));
